simulink model "SRAM"  (R2022a)
settings: Solver=VariableStepAuto  StartTime=0.0  StopTime=50  RelTol=1e-3
libraries: simulink x6, hdlsllib x2
settings Model: Creator=abhig  LastModifiedBy=abhig

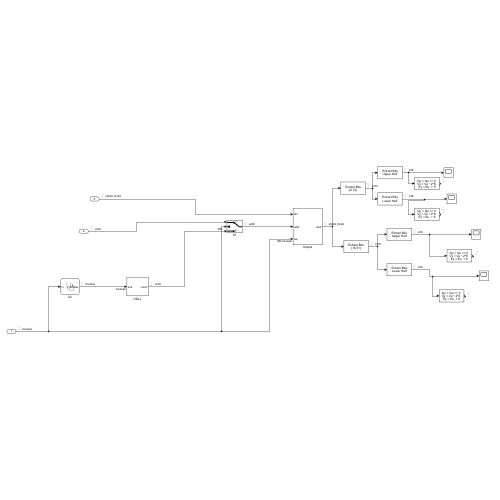
[thumbnail: Simulink's stored preview of the top-level diagram]
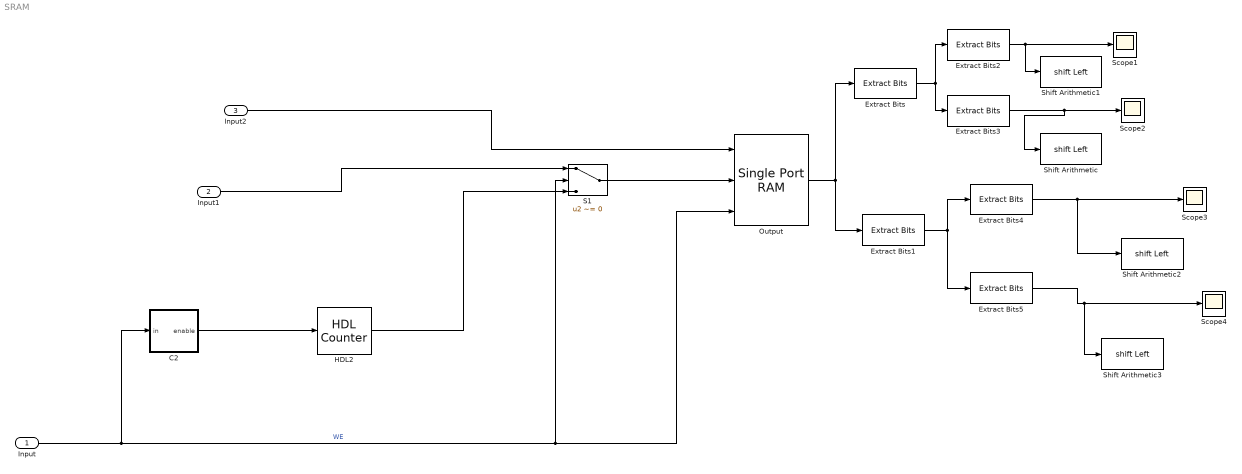
== system SRAM ==
  Input : Inport  OutDataTypeStr=boolean
  Input1 : Inport  Port=2
  Input2 : Inport  Port=3  OutDataTypeStr=fixdt(1,32,24)
  C2 : Stateflow chart  TreatAsAtomicUnit=on
  Extract Bits : simulink/Logic and Bit Operations/Extract Bits  bitsToExtract=Range of bits  numBits=8  bitIdxRange=[0 15]  outScalingMode=Treat bit field as an integer
  Extract Bits1 : simulink/Logic and Bit Operations/Extract Bits  bitsToExtract=Range of bits  numBits=8  bitIdxRange=[16 31]  outScalingMode=Treat bit field as an integer
  Extract Bits2 : simulink/Logic and Bit Operations/Extract Bits  bitsToExtract=Upper half  numBits=8  bitIdxRange=[15 8]  outScalingMode=Treat bit field as an integer
  Extract Bits3 : simulink/Logic and Bit Operations/Extract Bits  bitsToExtract=Lower half  numBits=8  bitIdxRange=[0 7]  outScalingMode=Treat bit field as an integer
  Extract Bits4 : simulink/Logic and Bit Operations/Extract Bits  bitsToExtract=Upper half  numBits=8  bitIdxRange=[15 8]  outScalingMode=Treat bit field as an integer
  Extract Bits5 : simulink/Logic and Bit Operations/Extract Bits  bitsToExtract=Lower half  numBits=8  bitIdxRange=[0 7]  outScalingMode=Treat bit field as an integer
  HDL2 : hdlsllib/Sources/HDL Counter  CountType=Count limited  CountInit=1  CountStep=1  CountMax=10  CountFromType=Initial value  CountFrom=1  CountResetPort=off  CountLoadPort=off  CountEnbPort=on  CountDirPort=off  CountHitOutputPort=off  CountDataType=Unsigned  CountWordLen=8  CountFracLen=0  CountSampTime=1
  Output : hdlsllib/HDL RAMs/Single Port RAM  ram_size=8  dout_type=New data
      settings: SourceProductBaseCode=SL
  S1 : Switch  Criteria=u2 ~= 0  SaturateOnIntegerOverflow=off  InputSameDT=off
  Scope{1..4} (4 alike) : Scope
  Shift Arithmetic{,1..3} (4 alike) : ArithShift  BinPtShiftNumber=6  BitShiftDirection=Left
  wires:
  Input/1 -> C2/1(in), S1/2, Output/3  "WE"
  S1/1 -> Output/2
  Output/1 -> Extract Bits1/1, Extract Bits/1
  Input1/1 -> S1/1
  Input2/1 -> Output/1
  HDL2/1 -> S1/3
  C2/1(enable) -> HDL2/1
  Extract Bits/1 -> Extract Bits3/1, Extract Bits2/1
  Extract Bits1/1 -> Extract Bits5/1, Extract Bits4/1
  Extract Bits2/1 -> Shift Arithmetic1/1, Scope1/1
  Extract Bits3/1 -> Shift Arithmetic/1, Scope2/1
  Extract Bits4/1 -> Shift Arithmetic2/1, Scope3/1
  Extract Bits5/1 -> Shift Arithmetic3/1, Scope4/1

== stateflow chart SRAM/C2 ==
  state default
    enable=true
  state add
    entry:x=0,enable=false;
    during :x=x+0.25;
  state x
    enable=false
  add -> x [order 2] : [in==1]
  (default) -> add
  default -> add [order 1] : [in==0]
  x -> add : [in==0]
  default -> x [order 2] : [in==1]
  add -> default [order 1] : [x>=0&&in==0]
  data: x local; enable output; in input
